simulink model "g1_G2_01"  (R2024a)
settings: Solver=ode1  StartTime=0.0  StopTime=0.3  FixedStep=Ts  RelTol=1e-3
PostLoadFcn:
  | GL_cbfcn('PostLoadFcn');
InitFcn:
  | GL_cbfcn('InitFcn');
StartFcn:
  | GL_cbfcn('StartFcn');
values from neighbouring files (symbols this model uses):
  Ts = 5e-4    (= 0.0005)    [g1_ini_01.m]    (also in g1_opam_ini_01.m; test.m = 0.001)
undefined symbols (not defined in the file or in its folder): burblks, DiscIntNeverNeededParam, GL_cbfcn
libraries: bur_blks x1
(part 1 of 2)
PreSaveFcn:
  | GL_cbfcn('PreSaveFcn');
PostSaveFcn:
  | GL_cbfcn('PostSaveFcn');
CloseFcn:
  | GL_cbfcn('CloseFcn');
settings Model: GhostLab=GhostLab  GhostLab_ModelName=Modular2  GhostLab_Version=2.0.4  CheckSum_Model=3251361011_3166437564_2525209146_3089150091  AS_Version=1.0.4  ExtModeTrigDuration=10000000  Creator=fldr  LastModifiedBy=rueegan5
settings DataIOCC: SaveFormat=Array  SaveOutput=off  SignalLogging=off  DSMLogging=off  SaveTime=off  ReturnWorkspaceOutputs=off
settings OptimizationCC: OptimizeBlockIOStorage=off  BufferReuse=off  GlobalBufferReuse=off  ExpressionFolding=off  EnableMemcpy=off  LocalBlockOutputs=off  InitFltsAndDblsToZero=on  LifeSpan=inf  OptimizeDataStoreBuffers=off  BusAssignmentInplaceUpdate=off
settings DebuggingCC: SaveWithDisabledLinksMsg=none  UnderspecifiedInitializationDetection=Classic  MergeDetectMultiDrivingBlocksExec=none  SolverPrmCheckMsg=warning  InheritedTsInSrcMsg=none  FcnCallInpInsideContextMsg=warning  FrameProcessingCompatibilityMsg=none  ModelReferenceSymbolNameMessage=none  StateNameClashWarn=warning  SFUnexpectedBacktrackingDiag=warning  SFNoUnconditionalDefaultTransitionDiag=warning
settings HardwareCC: ProdBitPerPointer=32  ProdBitPerSizeT=32  ProdBitPerPtrDiffT=32  ProdLargestAtomicFloat=None  ProdWordSize=32  ProdHWDeviceType=Intel->x86/Pentium
settings ModelReferenceCC: UpdateModelReferenceTargets=IfOutOfDate  ModelReferencePassRootInputsByReference=off  PropagateSignalLabelsOutOfModel=off
settings RTWCC: Description=B&R Automation Studio Target (GRT based)  SystemTargetFile=bur_grt.tlc  GenerateMakefile=off  TemplateMakefile=bur.tmf  RTWVerbose=off
settings RTWCC: CustomInitializer=|
  | udCheckSum0 = (0123456789U);
  | udCheckSum1 = (0123456789U);
  | udCheckSum2 = (0123456789U);
  | udCheckSum3 = (0123456789U);
  | udCurrentTime = &g1_G2_01_M->Timing.t[0];
  | udclockTick0 = &g1_G2_01_M->Timing.clockTick0;
  | udclockTickH0 = &g1_G2_01_M->Timing.clockTickH0;
  | udParam = &g1_G2_01_P;
  | udContinuousStates = &g1_G2_01_X;
  | udDiscreteStates = &g1_G2_01_DW;
settings CodeAppCC: MaxIdLength=255
settings STFCustomTargetCC: TargetLangStandard=C89/C90 (ANSI)  ParMdlRefBuildCompliant=on  UseToolchainInfoCompliant=off  SystemTargetFile=bur_grt.tlc
settings GRTTargetCC: TargetLangStandard=C89/C90 (ANSI)  CompOptLevelCompliant=off  ConcurrentExecutionCompliant=off  CombineOutputUpdateFcns=off  MatFileLogging=off  CPPClassGenCompliant=off  GRTInterface=on  UseToolchainInfoCompliant=off  ExtModeMexArgs='127.0.0.1'

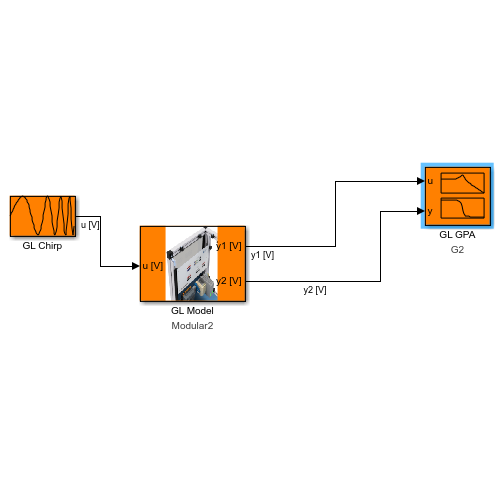
[thumbnail: Simulink's stored preview of the top-level diagram]
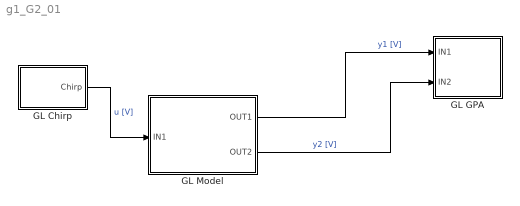
== system g1_G2_01 ==
  GL Chirp : Subsystem  LoadFcn=GL_cbfcn('loadChirp');  InitFcn=GL_cbfcn('initChirp');  mask(GhostLab Chirp){mode=logarithmic, f1=0.1, f2=1000, ampl=1, offs=0, T0=0, Tm=10, editSweepTime=off, Trig=1, mode_n=2, Dummy=0}
      mask prompts: mode "Sweep Sine Mode"; f1 "Start Frequency [Hz]"; f2 "End Frequency [Hz]"; ampl "Amplitude"; offs "Offset"; T0 "Settle Time [s]"; Tm "Sweep Time [s]"; editSweepTime "Edit"; Trig "Trigger"; mode_n "Chirp Mode"
      mask help: Creates a chirp (sweep sinus) signal used for gain phase analyzer.
      settings: CopyFcn=GL_cbfcn('copyChirp');  PreCopyFcn=GL_cbfcn('PreCopyChirp');
      mask Help: 1.0.2
      mask TypeOptions mode: linear | logarithmic | quadratic
      mask Callback mode:
      | try
      |     GL_cbfcn('ChirpMode');
      | end
      mask Callback f1:
      | try
      |     GL_cbfcn('fstart');
      | end
      | try
      |     GL_cbfcn('editSweepTime');
      | end
      mask Callback f2:
      | try
      |     GL_cbfcn('fend');
      | end
      mask Callback ampl:
      | try
      |     GL_cbfcn('ApplyChanges');
      | end
      mask Callback offs:
      | try
      |     GL_cbfcn('ApplyChanges');
      | end
      mask Callback T0:
      | try
      |     GL_cbfcn('ApplyChanges');
      | end
      mask Callback Tm:
      | try
      |     GL_cbfcn('ApplyChanges');
      | end
      mask Callback editSweepTime:
      | try
      |     GL_cbfcn('editSweepTime');
      | end
      mask DialogControl DescGroupVar Prompt: Chirp Signal Generator
      mask Display: plot(chirp(0:0.1:10,0.1,10,1,'logarithmic',-90));
  GL GPA : Subsystem  Tag=G2  Description=GL_cbfcn('openMask');  mask(GhostLab GPA){varname=G2}
      mask prompts: varname "Workspace Variable Name:"
      mask help:
      | Calculate and plot bode diagram using tfestimate.
      | An FRD-object and a structure with time data variable will be created in worspace.
      settings: AttributesFormatString=%<Tag>  CopyFcn=GL_cbfcn('copyGPA',gcb,'G');  DeleteFcn=GL_cbfcn('deleteScope');  UndoDeleteFcn=GL_cbfcn('updateScope');  PreCopyFcn=GL_cbfcn('PreCopyGPA');  OpenFcn=GL_cbfcn('openMask');
      mask Help: 1.0.2
      mask Callback varname: GL_cbfcn('set_var_name');
      mask DialogControl DescGroupVar Prompt: Gain Phase Analyzer
      mask DialogControl Control2 Prompt: help tfetimate
      mask DialogControl Control2 Callback: doc('tfestimate');
      mask DialogControl Container2 Prompt: Frequency Response Data (FRD) object:
      mask Display:
      | mat = [
      |    10.0000   78.3832   42.8007
      |    11.6327   78.3936   42.7806
      |    13.2653   78.4061   42.7584
      |    14.8980   78.4213   42.7338
      |    16.5306   78.4397   42.7064
      |    18.1633   78.4620   42.6761
      |    19.7959   78.4890   42.6423
      |    21.4286   78.5217   42.6044
      |    23.0612   78.5616   42.5620
      |    24.6939   78.6100   42.5142
      |    26.3265   78.6691   42.4600
      |    27.9592   78.7412   42.3982
      |    29.5918   78.8296   42.3272
      |    31.2245   78.9383   42.2447
      |    32.8571   79.0724   42.1478
      |    34.4898   79.2389   42.0322
      |    36.1224   79.4469   41.8917
      |    37.7551   79.7090   41.7169
      |    39.3878   80.0430   41.4928
      |    41.0204   80.4749   41.1939
      |    42.6531   81.0442   40.7735
      |    44.2857   81.8142   40.1368
      |    45.9184   82.8890   39.0620
      |    47.5510   84.4186   36.9274
      |    49.1837   86.2203   31.8362
      |    50.8163   85.7441   23.1638
      |    52.4490   82.9900   18.0726
      |    54.0816   80.5081   15.9380
      |    55.7143   78.4809   14.8632
      |    57.3469   76.7585   14.2265
      |    58.9796   75.2368   13.8061
      |    60.6122   73.8525   13.5072
      |    62.2449   72.5661   13.2831
      |    63.8776   71.3516   13.1083
      |    65.5102   70.1913   12.9678
      |    67.1429   69.0724   12.8522
      |    68.7755   67.9859   12.7553
      |    70.4082   66.9248   12.6728
      |    72.0408   65.8841   12.6018
      |    73.6735   64.8595   12.5400
      |    75.3061   63.8481   12.4858
      |    76.9388   62.8473   12.4380
      |    78.5714   61.8551   12.3956
      |    80.2041   60.8699   12.3577
      |    81.8367   59.8905   12.3239
      |    83.4694   58.9159   12.2936
      |    85.1020   57.9451   12.2662
      |    86.7347   56.9776   12.2416
      |    88.3673   56.0126   12.2194
      |    90.0000   55.0499   12.1993
      | ];
      | plot(-20,0,...
      |     100,100,...
      |     [10,90,90,10,10], [45,45,10,10,45],...
      |     [10,90,90,10,10], [90,90,55,55,90],...
      |     mat(:,1),mat(:,2),mat(:,1),mat(:,3));
      | port_label('input', 1, 'u');
      | port_label('input', 2, 'y');
  GL Model : Subsystem  Tag=Modular2  Description=GL_SetupModel;  mask(GhostLab Model){}
      settings: AttributesFormatString=%<Tag>  CopyFcn=GL_CopyFcn;  DeleteFcn=GL_cbfcn('Blk_DeleteFcn');  UndoDeleteFcn=GL_CopyFcn('BoW');  PreCopyFcn=GL_cbfcn('Blk_PreCopyFcn');  OpenFcn=GL_SetupModel;
      mask Display: image('Modular2.png',[0.25,0,0.5,1]);color('black');port_label('input', 1, 'u [V]');port_label('output', 1, 'y1 [V]');port_label('output', 2, 'y2 [V]');
  wires:
  GL Chirp/1(Chirp) -> GL Model/1(IN1)  "u [V]"
  GL Model/1(OUT1) -> GL GPA/1(IN1)  "y1 [V]"
  GL Model/2(OUT2) -> GL GPA/2(IN2)  "y2 [V]"

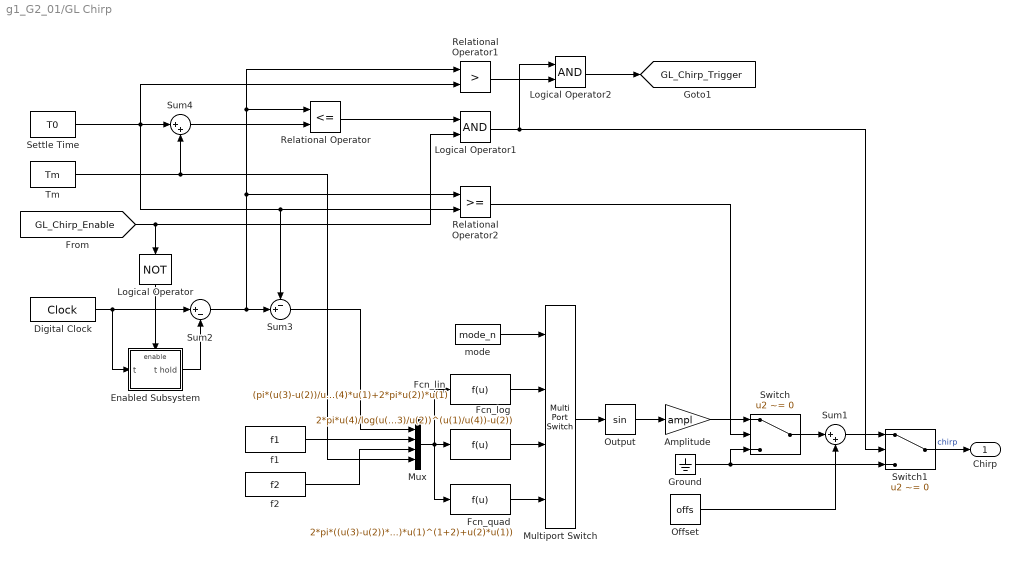
== system g1_G2_01/GL Chirp ==
  Amplitude : Gain  Gain=ampl
  Digital Clock : DigitalClock  SampleTime=Ts
  Enabled Subsystem : Subsystem  TreatAsAtomicUnit=on
  Fcn_lin : Fcn  Expr=(pi*(u(3)-u(2))/u(4)*u(1)+2*pi*u(2))*u(1)
  Fcn_log : Fcn  Expr=2*pi*u(4)/log(u(3)/u(2))*(u(2)*(u(3)/u(2))^(u(1)/u(4))-u(2))
  Fcn_quad : Fcn  Expr=2*pi*((u(3)-u(2))*u(4)^(-2)/(1+2)*u(1)^(1+2)+u(2)*u(1))
  Ground : Ground
  Logical Operator : Logic  Operator=NOT  AllPortsSameDT=off  OutDataTypeStr=boolean
  Logical Operator1 : Logic  AllPortsSameDT=off
  Logical Operator2 : Logic  AllPortsSameDT=off  OutDataTypeStr=boolean
  Multiport Switch : MultiPortSwitch  SaturateOnIntegerOverflow=off  InputSameDT=off
  Mux : Mux
  Offset : Constant  Value=offs
  Output : Trigonometry
  Relational Operator : RelationalOperator  Operator=<=  RndMeth=Simplest  InputSameDT=off
  Relational Operator1 : RelationalOperator  Operator=>  RndMeth=Simplest  InputSameDT=off
  Relational Operator2 : RelationalOperator  RndMeth=Simplest  InputSameDT=off
  Settle Time : Constant  Value=T0
  Sum1 : Sum  Inputs=|++
  Sum2 : Sum  Inputs=|+-
  Sum3 : Sum  Inputs=-+|
  Sum4 : Sum  Inputs=|++
  Switch : Switch  Criteria=u2 ~= 0  SaturateOnIntegerOverflow=off  InputSameDT=off
  Switch1 : Switch  Criteria=u2 ~= 0  SaturateOnIntegerOverflow=off  InputSameDT=off
  Tm : Constant  Value=Tm
  f1 : Constant  Value=f1
  f2 : Constant  Value=f2
  mode : Constant  Value=mode_n
  Chirp : Outport  VectorParamsAs1DForOutWhenUnconnected=off
  tag scope: GL_Chirp_Trigger=global
  wires:
  Relational Operator2/1 -> Switch/2
  Settle Time/1 -> Sum4/1, Relational Operator2/2, Sum3/1, Relational Operator1/2
  Sum4/1 -> Relational Operator/2
  Logical Operator/1 -> Enabled Subsystem/Enable
  Enabled Subsystem/1(t hold) -> Sum2/2
  [GL_Chirp_Enable] -> Logical Operator1/2, Logical Operator/1
  mode/1 -> Multiport Switch/1
  Fcn_lin/1 -> Multiport Switch/2
  Fcn_log/1 -> Multiport Switch/3
  Fcn_quad/1 -> Multiport Switch/4
  Multiport Switch/1 -> Output/1
  f2/1 -> Mux/3
  f1/1 -> Mux/2
  Mux/1 -> Fcn_log/1, Fcn_lin/1, Fcn_quad/1
  Output/1 -> Amplitude/1
  Offset/1 -> Sum1/2
  Sum3/1 -> Mux/1
  Tm/1 -> Sum4/2, Mux/4
  Switch/1 -> Sum1/1
  Amplitude/1 -> Switch/1
  Ground/1 -> Switch1/3, Switch/3
  Sum2/1 -> Relational Operator1/1, Relational Operator/1, Relational Operator2/1, Sum3/2
  Switch1/1 -> Chirp/1  "chirp"
  Sum1/1 -> Switch1/1
  Relational Operator/1 -> Logical Operator1/1
  Logical Operator1/1 -> Logical Operator2/1, Switch1/2
  Logical Operator2/1 -> [GL_Chirp_Trigger]
  Relational Operator1/1 -> Logical Operator2/2
  Digital Clock/1 -> Enabled Subsystem/1(t), Sum2/1

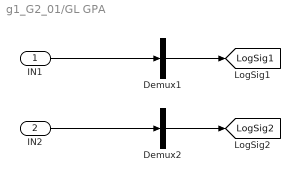
== system g1_G2_01/GL GPA ==
  IN1 : Inport
  IN2 : Inport  Port=2
  Demux1 : Demux  Outputs=1
  Demux2 : Demux  Outputs=1
  tag scope: LogSig1=global, LogSig2=global
  wires:
  IN2/1 -> Demux2/1
  IN1/1 -> Demux1/1
  Demux1/1 -> [LogSig1]
  Demux2/1 -> [LogSig2]

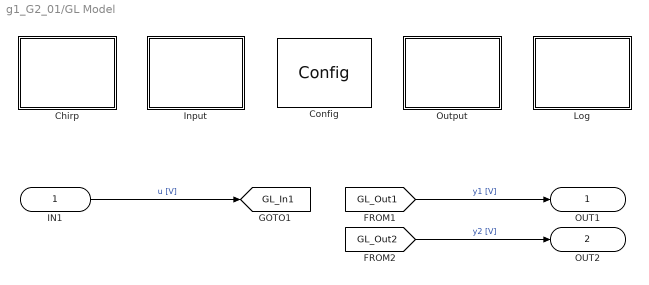
== system g1_G2_01/GL Model ==
  IN1 : Inport
  Chirp : Subsystem
  Config : bur_blks/Config  Tag=Coder: GRT C Target: Task  Description=burblks.classes.blks.BR_ConfigBlock.Do('open', gcb);  bur_configset_ert=C - Code Generation (Embedded Real Time Target based)  bur_configset_grt=C - Code Generation (Generic Real Time Target based)  bur_maskHandle=-1
      settings: AttributesFormatString=%<Tag>  SourceProductName=B&R Automation Studio Toolbox
  Input : Subsystem
  Log : Subsystem
  Output : Subsystem
  OUT1 : Outport
  OUT2 : Outport  Port=2
  tag scope: GL_In1=global
  wires:
  IN1/1 -> [GL_In1]  "u [V]"
  [GL_Out1] -> OUT1/1  "y1 [V]"
  [GL_Out2] -> OUT2/1  "y2 [V]"

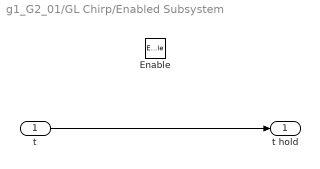
== system g1_G2_01/GL Chirp/Enabled Subsystem ==
  t : Inport
  Enable : EnablePort
  t hold : Outport  VectorParamsAs1DForOutWhenUnconnected=off
  wires:
  t/1 -> t hold/1

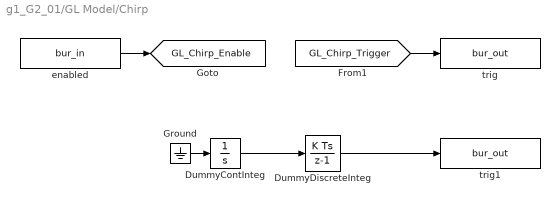
== system g1_G2_01/GL Model/Chirp ==
  DummyContInteg : Integrator
  DummyDiscreteInteg : DiscreteIntegrator  SampleTime=-1  OutDataTypeStr=single  ICPrevOutput=DiscIntNeverNeededParam  ICPrevScaledInput=DiscIntNeverNeededParam
  Ground : Ground
  enabled : S-Function  Tag=GLOBAL BOOL bConnectionEstablished  Description=burblks.classes.blks.BR_InputBlock.Do('open', gcb)  LoadFcn=burblks.classes.blks.BR_InputBlock.Do( 'load', gcb)  InitFcn=burblks.classes.blks.BR_InputBlock.Do('init', gcb)  FunctionName=bur_in  Parameters=bur_scope, bur_data_type, bur_init_value, bur_init_value_bool, bur_array_index, bur_var_name, bur_AS_string  SFunctionDeploymentMode=off  EnableBusSupport=off  mask(B&&R - Input Block){bur_var_name=bConnectionEstablished, bur_var_description=, bur_scope=GLOBAL, bur_data_type=BOOL, bur_init_value=0, bur_init_value_bool=FALSE, bur_array_index=0, bur_old_var_name=, bur_var_memory=standard, bur_in_parameter=off, bur_AS_string=bConnectionEstablished : BOOL := 0; (**), bur_array_index_string=0}
      mask prompts: bur_var_name "Variable Name"; bur_var_description "Variable Description"; bur_scope "Variable Scope"; bur_data_type "Variable Data Type"; bur_init_value "Initial Value"; bur_init_value_bool "Initial Value"; bur_array_index "Array Dimension (0...Scalar)"; bur_old_var_name "Old Variable Name"; bur_var_memory "Memory"; bur_in_parameter "Parameter"; bur_array_index_string "Array Dimension Variable (0..Scalar)"
      mask help: Input interface for B&R Automation Studio process variable.
      settings: AttributesFormatString=%<Tag>  CopyFcn=burblks.classes.blks.BR_InputBlock.Do('copy', gcb)  DeleteFcn=burblks.classes.blks.BR_InputBlock.Do( 'delete', gcb)  ModelCloseFcn=burblks.classes.blks.BR_InputBlock.Do('close', gcb)  PreSaveFcn=burblks.classes.blks.BR_InputBlock.Do('preSave', gcb)  PostSaveFcn=burblks.classes.blks.BR_InputBlock.Do('postSave', gcb)  OpenFcn=burblks.classes.blks.BR_InputBlock.Do('open', gcb)
      mask Help: eval('burblks.classes.blks.BR_BlockHelp.Help(''InputBlock'')')
      mask TypeOptions bur_scope: GLOBAL | LOCAL
      mask TypeOptions bur_data_type: LREAL | REAL | SINT | USINT | INT | UINT | DINT | UDINT | BOOL | STRING
      mask TypeOptions bur_init_value_bool: FALSE | TRUE
      mask TypeOptions bur_var_memory: standard | retain
      mask Display: color('orange'); disp('B&R IN');
  trig : S-Function  Tag=GLOBAL BOOL bGPAtrigger  Description=burblks.classes.blks.BR_OutputBlock.Do('open', gcb)  LoadFcn=burblks.classes.blks.BR_OutputBlock.Do( 'load', gcb)  InitFcn=burblks.classes.blks.BR_OutputBlock.Do('init', gcb)  FunctionName=bur_out  Parameters=bur_scope, bur_data_type, bur_init_value, bur_init_value_bool, bur_array_index, bur_var_name, bur_AS_string  SFunctionDeploymentMode=off  EnableBusSupport=off  mask(B&&R - Output Block){bur_var_name=bGPAtrigger, bur_var_description=, bur_scope=GLOBAL, bur_data_type=BOOL, bur_init_value=0, bur_init_value_bool=FALSE, bur_array_index=0, bur_old_var_name=, bur_var_memory=standard, bur_AS_string=bGPAtrigger : BOOL := 0; (**), bur_array_index_string=0}
      mask prompts: bur_var_name "Variable Name"; bur_var_description "Variable Description"; bur_scope "Variable Scope"; bur_data_type "Variable Data Type"; bur_init_value "Initial Value"; bur_init_value_bool "Initial Value"; bur_array_index "Array Dimension (0...Scalar)"; bur_old_var_name "Old Variable Name"; bur_var_memory "Memory"; bur_array_index_string "Array Dimension Variable (0..Scalar)"
      mask help: Output interface for B&R Automation Studio process variable.
      settings: AttributesFormatString=%<Tag>  CopyFcn=burblks.classes.blks.BR_OutputBlock.Do('copy', gcb)  DeleteFcn=burblks.classes.blks.BR_OutputBlock.Do( 'delete', gcb)  ModelCloseFcn=burblks.classes.blks.BR_OutputBlock.Do('close', gcb)  PreSaveFcn=burblks.classes.blks.BR_OutputBlock.Do('preSave', gcb)  PostSaveFcn=burblks.classes.blks.BR_OutputBlock.Do('postSave', gcb)  OpenFcn=burblks.classes.blks.BR_OutputBlock.Do('open', gcb)
      mask Help: eval('burblks.classes.blks.BR_BlockHelp.Help(''OutputBlock'')')
      mask TypeOptions bur_scope: GLOBAL | LOCAL
      mask TypeOptions bur_data_type: LREAL | REAL | SINT | USINT | INT | UINT | DINT | UDINT | BOOL | STRING
      mask TypeOptions bur_init_value_bool: FALSE | TRUE
      mask TypeOptions bur_var_memory: standard | retain
      mask Display: color('orange'); disp('B&R OUT');
  trig1 : S-Function  Tag=GLOBAL REAL rDummy  Description=burblks.classes.blks.BR_OutputBlock.Do('open', gcb)  LoadFcn=burblks.classes.blks.BR_OutputBlock.Do( 'load', gcb)  InitFcn=burblks.classes.blks.BR_OutputBlock.Do('init', gcb)  FunctionName=bur_out  Parameters=bur_scope, bur_data_type, bur_init_value, bur_init_value_bool, bur_array_index, bur_var_name, bur_AS_string  SFunctionDeploymentMode=off  EnableBusSupport=off  mask(B&&R - Output Block){bur_var_name=rDummy, bur_var_description=, bur_scope=GLOBAL, bur_data_type=REAL, bur_init_value=0, bur_init_value_bool=FALSE, bur_array_index=0, bur_old_var_name=, bur_var_memory=standard, bur_AS_string=rDummy : REAL := 0; (**), bur_array_index_string=0}
      mask prompts: bur_var_name "Variable Name"; bur_var_description "Variable Description"; bur_scope "Variable Scope"; bur_data_type "Variable Data Type"; bur_init_value "Initial Value"; bur_init_value_bool "Initial Value"; bur_array_index "Array Dimension (0...Scalar)"; bur_old_var_name "Old Variable Name"; bur_var_memory "Memory"; bur_array_index_string "Array Dimension Variable (0..Scalar)"
      mask help: Output interface for B&R Automation Studio process variable.
      settings: AttributesFormatString=%<Tag>  CopyFcn=burblks.classes.blks.BR_OutputBlock.Do('copy', gcb)  DeleteFcn=burblks.classes.blks.BR_OutputBlock.Do( 'delete', gcb)  ModelCloseFcn=burblks.classes.blks.BR_OutputBlock.Do('close', gcb)  PreSaveFcn=burblks.classes.blks.BR_OutputBlock.Do('preSave', gcb)  PostSaveFcn=burblks.classes.blks.BR_OutputBlock.Do('postSave', gcb)  OpenFcn=burblks.classes.blks.BR_OutputBlock.Do('open', gcb)
      mask Help: eval('burblks.classes.blks.BR_BlockHelp.Help(''OutputBlock'')')
      mask TypeOptions bur_scope: GLOBAL | LOCAL
      mask TypeOptions bur_data_type: LREAL | REAL | SINT | USINT | INT | UINT | DINT | UDINT | BOOL | STRING
      mask TypeOptions bur_init_value_bool: FALSE | TRUE
      mask TypeOptions bur_var_memory: standard | retain
      mask Display: color('orange'); disp('B&R OUT');
  tag scope: GL_Chirp_Enable=global
  wires:
  [GL_Chirp_Trigger] -> trig/1
  enabled/1 -> [GL_Chirp_Enable]
  DummyContInteg/1 -> DummyDiscreteInteg/1
  Ground/1 -> DummyContInteg/1
  DummyDiscreteInteg/1 -> trig1/1

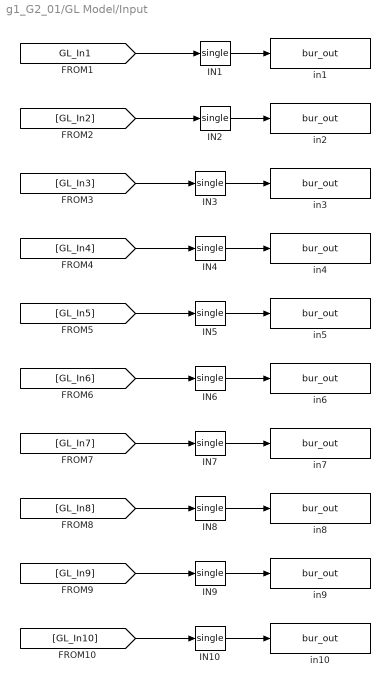
== system g1_G2_01/GL Model/Input ==
  IN{1..10} (10 alike) : DataTypeConversion  OutDataTypeStr=single  SaturateOnIntegerOverflow=off  RndMeth=Floor
  in1 : S-Function  Tag=GLOBAL REAL rSimInput1  Description=burblks.classes.blks.BR_OutputBlock.Do('open', gcb)  LoadFcn=burblks.classes.blks.BR_OutputBlock.Do( 'load', gcb)  InitFcn=burblks.classes.blks.BR_OutputBlock.Do('init', gcb)  FunctionName=bur_out  Parameters=bur_scope, bur_data_type, bur_init_value, bur_init_value_bool, bur_array_index, bur_var_name, bur_AS_string  SFunctionDeploymentMode=off  EnableBusSupport=off  mask(B&&R - Output Block){bur_var_name=rSimInput1, bur_var_description=, bur_scope=GLOBAL, bur_data_type=REAL, bur_init_value=0, bur_init_value_bool=FALSE, bur_array_index=0, bur_old_var_name=, bur_var_memory=standard, bur_AS_string=rSimInput1 : REAL := 0; (**), bur_array_index_string=0}
      mask prompts: bur_var_name "Variable Name"; bur_var_description "Variable Description"; bur_scope "Variable Scope"; bur_data_type "Variable Data Type"; bur_init_value "Initial Value"; bur_init_value_bool "Initial Value"; bur_array_index "Array Dimension (0...Scalar)"; bur_old_var_name "Old Variable Name"; bur_var_memory "Memory"; bur_array_index_string "Array Dimension Variable (0..Scalar)"
      mask help: Output interface for B&R Automation Studio process variable.
      settings: AttributesFormatString=%<Tag>  CopyFcn=burblks.classes.blks.BR_OutputBlock.Do('copy', gcb)  DeleteFcn=burblks.classes.blks.BR_OutputBlock.Do( 'delete', gcb)  ModelCloseFcn=burblks.classes.blks.BR_OutputBlock.Do('close', gcb)  PreSaveFcn=burblks.classes.blks.BR_OutputBlock.Do('preSave', gcb)  PostSaveFcn=burblks.classes.blks.BR_OutputBlock.Do('postSave', gcb)  OpenFcn=burblks.classes.blks.BR_OutputBlock.Do('open', gcb)
      mask Help: eval('burblks.classes.blks.BR_BlockHelp.Help(''OutputBlock'')')
      mask TypeOptions bur_scope: GLOBAL | LOCAL
      mask TypeOptions bur_data_type: LREAL | REAL | SINT | USINT | INT | UINT | DINT | UDINT | BOOL | STRING
      mask TypeOptions bur_init_value_bool: FALSE | TRUE
      mask TypeOptions bur_var_memory: standard | retain
      mask Display: color('orange'); disp('B&R OUT');
  in10 : S-Function  Tag=GLOBAL REAL rSimInput10  Description=burblks.classes.blks.BR_OutputBlock.Do('open', gcb)  LoadFcn=burblks.classes.blks.BR_OutputBlock.Do( 'load', gcb)  InitFcn=burblks.classes.blks.BR_OutputBlock.Do('init', gcb)  FunctionName=bur_out  Parameters=bur_scope, bur_data_type, bur_init_value, bur_init_value_bool, bur_array_index, bur_var_name, bur_AS_string  SFunctionDeploymentMode=off  EnableBusSupport=off  mask(B&&R - Output Block){bur_var_name=rSimInput10, bur_var_description=, bur_scope=GLOBAL, bur_data_type=REAL, bur_init_value=0, bur_init_value_bool=FALSE, bur_array_index=0, bur_old_var_name=, bur_var_memory=standard, bur_AS_string=rSimInput10 : REAL := 0; (**), bur_array_index_string=0}
      mask prompts: bur_var_name "Variable Name"; bur_var_description "Variable Description"; bur_scope "Variable Scope"; bur_data_type "Variable Data Type"; bur_init_value "Initial Value"; bur_init_value_bool "Initial Value"; bur_array_index "Array Dimension (0...Scalar)"; bur_old_var_name "Old Variable Name"; bur_var_memory "Memory"; bur_array_index_string "Array Dimension Variable (0..Scalar)"
      mask help: Output interface for B&R Automation Studio process variable.
      settings: AttributesFormatString=%<Tag>  CopyFcn=burblks.classes.blks.BR_OutputBlock.Do('copy', gcb)  DeleteFcn=burblks.classes.blks.BR_OutputBlock.Do( 'delete', gcb)  ModelCloseFcn=burblks.classes.blks.BR_OutputBlock.Do('close', gcb)  PreSaveFcn=burblks.classes.blks.BR_OutputBlock.Do('preSave', gcb)  PostSaveFcn=burblks.classes.blks.BR_OutputBlock.Do('postSave', gcb)  OpenFcn=burblks.classes.blks.BR_OutputBlock.Do('open', gcb)
      mask Help: eval('burblks.classes.blks.BR_BlockHelp.Help(''OutputBlock'')')
      mask TypeOptions bur_scope: GLOBAL | LOCAL
      mask TypeOptions bur_data_type: LREAL | REAL | SINT | USINT | INT | UINT | DINT | UDINT | BOOL | STRING
      mask TypeOptions bur_init_value_bool: FALSE | TRUE
      mask TypeOptions bur_var_memory: standard | retain
      mask Display: color('orange'); disp('B&R OUT');
  in2 : S-Function  Tag=GLOBAL REAL rSimInput2  Description=burblks.classes.blks.BR_OutputBlock.Do('open', gcb)  LoadFcn=burblks.classes.blks.BR_OutputBlock.Do( 'load', gcb)  InitFcn=burblks.classes.blks.BR_OutputBlock.Do('init', gcb)  FunctionName=bur_out  Parameters=bur_scope, bur_data_type, bur_init_value, bur_init_value_bool, bur_array_index, bur_var_name, bur_AS_string  SFunctionDeploymentMode=off  EnableBusSupport=off  mask(B&&R - Output Block){bur_var_name=rSimInput2, bur_var_description=, bur_scope=GLOBAL, bur_data_type=REAL, bur_init_value=0, bur_init_value_bool=FALSE, bur_array_index=0, bur_old_var_name=, bur_var_memory=standard, bur_AS_string=rSimInput2 : REAL := 0; (**), bur_array_index_string=0}
      mask prompts: bur_var_name "Variable Name"; bur_var_description "Variable Description"; bur_scope "Variable Scope"; bur_data_type "Variable Data Type"; bur_init_value "Initial Value"; bur_init_value_bool "Initial Value"; bur_array_index "Array Dimension (0...Scalar)"; bur_old_var_name "Old Variable Name"; bur_var_memory "Memory"; bur_array_index_string "Array Dimension Variable (0..Scalar)"
      mask help: Output interface for B&R Automation Studio process variable.
      settings: AttributesFormatString=%<Tag>  CopyFcn=burblks.classes.blks.BR_OutputBlock.Do('copy', gcb)  DeleteFcn=burblks.classes.blks.BR_OutputBlock.Do( 'delete', gcb)  ModelCloseFcn=burblks.classes.blks.BR_OutputBlock.Do('close', gcb)  PreSaveFcn=burblks.classes.blks.BR_OutputBlock.Do('preSave', gcb)  PostSaveFcn=burblks.classes.blks.BR_OutputBlock.Do('postSave', gcb)  OpenFcn=burblks.classes.blks.BR_OutputBlock.Do('open', gcb)
      mask Help: eval('burblks.classes.blks.BR_BlockHelp.Help(''OutputBlock'')')
      mask TypeOptions bur_scope: GLOBAL | LOCAL
      mask TypeOptions bur_data_type: LREAL | REAL | SINT | USINT | INT | UINT | DINT | UDINT | BOOL | STRING
      mask TypeOptions bur_init_value_bool: FALSE | TRUE
      mask TypeOptions bur_var_memory: standard | retain
      mask Display: color('orange'); disp('B&R OUT');
  in3 : S-Function  Tag=GLOBAL REAL rSimInput3  Description=burblks.classes.blks.BR_OutputBlock.Do('open', gcb)  LoadFcn=burblks.classes.blks.BR_OutputBlock.Do( 'load', gcb)  InitFcn=burblks.classes.blks.BR_OutputBlock.Do('init', gcb)  FunctionName=bur_out  Parameters=bur_scope, bur_data_type, bur_init_value, bur_init_value_bool, bur_array_index, bur_var_name, bur_AS_string  SFunctionDeploymentMode=off  EnableBusSupport=off  mask(B&&R - Output Block){bur_var_name=rSimInput3, bur_var_description=, bur_scope=GLOBAL, bur_data_type=REAL, bur_init_value=0, bur_init_value_bool=FALSE, bur_array_index=0, bur_old_var_name=, bur_var_memory=standard, bur_AS_string=rSimInput3 : REAL := 0; (**), bur_array_index_string=0}
      mask prompts: bur_var_name "Variable Name"; bur_var_description "Variable Description"; bur_scope "Variable Scope"; bur_data_type "Variable Data Type"; bur_init_value "Initial Value"; bur_init_value_bool "Initial Value"; bur_array_index "Array Dimension (0...Scalar)"; bur_old_var_name "Old Variable Name"; bur_var_memory "Memory"; bur_array_index_string "Array Dimension Variable (0..Scalar)"
      mask help: Output interface for B&R Automation Studio process variable.
      settings: AttributesFormatString=%<Tag>  CopyFcn=burblks.classes.blks.BR_OutputBlock.Do('copy', gcb)  DeleteFcn=burblks.classes.blks.BR_OutputBlock.Do( 'delete', gcb)  ModelCloseFcn=burblks.classes.blks.BR_OutputBlock.Do('close', gcb)  PreSaveFcn=burblks.classes.blks.BR_OutputBlock.Do('preSave', gcb)  PostSaveFcn=burblks.classes.blks.BR_OutputBlock.Do('postSave', gcb)  OpenFcn=burblks.classes.blks.BR_OutputBlock.Do('open', gcb)
      mask Help: eval('burblks.classes.blks.BR_BlockHelp.Help(''OutputBlock'')')
      mask TypeOptions bur_scope: GLOBAL | LOCAL
      mask TypeOptions bur_data_type: LREAL | REAL | SINT | USINT | INT | UINT | DINT | UDINT | BOOL | STRING
      mask TypeOptions bur_init_value_bool: FALSE | TRUE
      mask TypeOptions bur_var_memory: standard | retain
      mask Display: color('orange'); disp('B&R OUT');
  in4 : S-Function  Tag=GLOBAL REAL rSimInput4  Description=burblks.classes.blks.BR_OutputBlock.Do('open', gcb)  LoadFcn=burblks.classes.blks.BR_OutputBlock.Do( 'load', gcb)  InitFcn=burblks.classes.blks.BR_OutputBlock.Do('init', gcb)  FunctionName=bur_out  Parameters=bur_scope, bur_data_type, bur_init_value, bur_init_value_bool, bur_array_index, bur_var_name, bur_AS_string  SFunctionDeploymentMode=off  EnableBusSupport=off  mask(B&&R - Output Block){bur_var_name=rSimInput4, bur_var_description=, bur_scope=GLOBAL, bur_data_type=REAL, bur_init_value=0, bur_init_value_bool=FALSE, bur_array_index=0, bur_old_var_name=, bur_var_memory=standard, bur_AS_string=rSimInput4 : REAL := 0; (**), bur_array_index_string=0}
      mask prompts: bur_var_name "Variable Name"; bur_var_description "Variable Description"; bur_scope "Variable Scope"; bur_data_type "Variable Data Type"; bur_init_value "Initial Value"; bur_init_value_bool "Initial Value"; bur_array_index "Array Dimension (0...Scalar)"; bur_old_var_name "Old Variable Name"; bur_var_memory "Memory"; bur_array_index_string "Array Dimension Variable (0..Scalar)"
      mask help: Output interface for B&R Automation Studio process variable.
      settings: AttributesFormatString=%<Tag>  CopyFcn=burblks.classes.blks.BR_OutputBlock.Do('copy', gcb)  DeleteFcn=burblks.classes.blks.BR_OutputBlock.Do( 'delete', gcb)  ModelCloseFcn=burblks.classes.blks.BR_OutputBlock.Do('close', gcb)  PreSaveFcn=burblks.classes.blks.BR_OutputBlock.Do('preSave', gcb)  PostSaveFcn=burblks.classes.blks.BR_OutputBlock.Do('postSave', gcb)  OpenFcn=burblks.classes.blks.BR_OutputBlock.Do('open', gcb)
      mask Help: eval('burblks.classes.blks.BR_BlockHelp.Help(''OutputBlock'')')
      mask TypeOptions bur_scope: GLOBAL | LOCAL
      mask TypeOptions bur_data_type: LREAL | REAL | SINT | USINT | INT | UINT | DINT | UDINT | BOOL | STRING
      mask TypeOptions bur_init_value_bool: FALSE | TRUE
      mask TypeOptions bur_var_memory: standard | retain
      mask Display: color('orange'); disp('B&R OUT');
  in5 : S-Function  Tag=GLOBAL REAL rSimInput5  Description=burblks.classes.blks.BR_OutputBlock.Do('open', gcb)  LoadFcn=burblks.classes.blks.BR_OutputBlock.Do( 'load', gcb)  InitFcn=burblks.classes.blks.BR_OutputBlock.Do('init', gcb)  FunctionName=bur_out  Parameters=bur_scope, bur_data_type, bur_init_value, bur_init_value_bool, bur_array_index, bur_var_name, bur_AS_string  SFunctionDeploymentMode=off  EnableBusSupport=off  mask(B&&R - Output Block){bur_var_name=rSimInput5, bur_var_description=, bur_scope=GLOBAL, bur_data_type=REAL, bur_init_value=0, bur_init_value_bool=FALSE, bur_array_index=0, bur_old_var_name=, bur_var_memory=standard, bur_AS_string=rSimInput5 : REAL := 0; (**), bur_array_index_string=0}
      mask prompts: bur_var_name "Variable Name"; bur_var_description "Variable Description"; bur_scope "Variable Scope"; bur_data_type "Variable Data Type"; bur_init_value "Initial Value"; bur_init_value_bool "Initial Value"; bur_array_index "Array Dimension (0...Scalar)"; bur_old_var_name "Old Variable Name"; bur_var_memory "Memory"; bur_array_index_string "Array Dimension Variable (0..Scalar)"
      mask help: Output interface for B&R Automation Studio process variable.
      settings: AttributesFormatString=%<Tag>  CopyFcn=burblks.classes.blks.BR_OutputBlock.Do('copy', gcb)  DeleteFcn=burblks.classes.blks.BR_OutputBlock.Do( 'delete', gcb)  ModelCloseFcn=burblks.classes.blks.BR_OutputBlock.Do('close', gcb)  PreSaveFcn=burblks.classes.blks.BR_OutputBlock.Do('preSave', gcb)  PostSaveFcn=burblks.classes.blks.BR_OutputBlock.Do('postSave', gcb)  OpenFcn=burblks.classes.blks.BR_OutputBlock.Do('open', gcb)
      mask Help: eval('burblks.classes.blks.BR_BlockHelp.Help(''OutputBlock'')')
      mask TypeOptions bur_scope: GLOBAL | LOCAL
      mask TypeOptions bur_data_type: LREAL | REAL | SINT | USINT | INT | UINT | DINT | UDINT | BOOL | STRING
      mask TypeOptions bur_init_value_bool: FALSE | TRUE
      mask TypeOptions bur_var_memory: standard | retain
      mask Display: color('orange'); disp('B&R OUT');
  in6 : S-Function  Tag=GLOBAL REAL rSimInput6  Description=burblks.classes.blks.BR_OutputBlock.Do('open', gcb)  LoadFcn=burblks.classes.blks.BR_OutputBlock.Do( 'load', gcb)  InitFcn=burblks.classes.blks.BR_OutputBlock.Do('init', gcb)  FunctionName=bur_out  Parameters=bur_scope, bur_data_type, bur_init_value, bur_init_value_bool, bur_array_index, bur_var_name, bur_AS_string  SFunctionDeploymentMode=off  EnableBusSupport=off  mask(B&&R - Output Block){bur_var_name=rSimInput6, bur_var_description=, bur_scope=GLOBAL, bur_data_type=REAL, bur_init_value=0, bur_init_value_bool=FALSE, bur_array_index=0, bur_old_var_name=, bur_var_memory=standard, bur_AS_string=rSimInput6 : REAL := 0; (**), bur_array_index_string=0}
      mask prompts: bur_var_name "Variable Name"; bur_var_description "Variable Description"; bur_scope "Variable Scope"; bur_data_type "Variable Data Type"; bur_init_value "Initial Value"; bur_init_value_bool "Initial Value"; bur_array_index "Array Dimension (0...Scalar)"; bur_old_var_name "Old Variable Name"; bur_var_memory "Memory"; bur_array_index_string "Array Dimension Variable (0..Scalar)"
      mask help: Output interface for B&R Automation Studio process variable.
      settings: AttributesFormatString=%<Tag>  CopyFcn=burblks.classes.blks.BR_OutputBlock.Do('copy', gcb)  DeleteFcn=burblks.classes.blks.BR_OutputBlock.Do( 'delete', gcb)  ModelCloseFcn=burblks.classes.blks.BR_OutputBlock.Do('close', gcb)  PreSaveFcn=burblks.classes.blks.BR_OutputBlock.Do('preSave', gcb)  PostSaveFcn=burblks.classes.blks.BR_OutputBlock.Do('postSave', gcb)  OpenFcn=burblks.classes.blks.BR_OutputBlock.Do('open', gcb)
      mask Help: eval('burblks.classes.blks.BR_BlockHelp.Help(''OutputBlock'')')
      mask TypeOptions bur_scope: GLOBAL | LOCAL
      mask TypeOptions bur_data_type: LREAL | REAL | SINT | USINT | INT | UINT | DINT | UDINT | BOOL | STRING
      mask TypeOptions bur_init_value_bool: FALSE | TRUE
      mask TypeOptions bur_var_memory: standard | retain
      mask Display: color('orange'); disp('B&R OUT');
  in7 : S-Function  Tag=GLOBAL REAL rSimInput7  Description=burblks.classes.blks.BR_OutputBlock.Do('open', gcb)  LoadFcn=burblks.classes.blks.BR_OutputBlock.Do( 'load', gcb)  InitFcn=burblks.classes.blks.BR_OutputBlock.Do('init', gcb)  FunctionName=bur_out  Parameters=bur_scope, bur_data_type, bur_init_value, bur_init_value_bool, bur_array_index, bur_var_name, bur_AS_string  SFunctionDeploymentMode=off  EnableBusSupport=off  mask(B&&R - Output Block){bur_var_name=rSimInput7, bur_var_description=, bur_scope=GLOBAL, bur_data_type=REAL, bur_init_value=0, bur_init_value_bool=FALSE, bur_array_index=0, bur_old_var_name=, bur_var_memory=standard, bur_AS_string=rSimInput7 : REAL := 0; (**), bur_array_index_string=0}
      mask prompts: bur_var_name "Variable Name"; bur_var_description "Variable Description"; bur_scope "Variable Scope"; bur_data_type "Variable Data Type"; bur_init_value "Initial Value"; bur_init_value_bool "Initial Value"; bur_array_index "Array Dimension (0...Scalar)"; bur_old_var_name "Old Variable Name"; bur_var_memory "Memory"; bur_array_index_string "Array Dimension Variable (0..Scalar)"
      mask help: Output interface for B&R Automation Studio process variable.
      settings: AttributesFormatString=%<Tag>  CopyFcn=burblks.classes.blks.BR_OutputBlock.Do('copy', gcb)  DeleteFcn=burblks.classes.blks.BR_OutputBlock.Do( 'delete', gcb)  ModelCloseFcn=burblks.classes.blks.BR_OutputBlock.Do('close', gcb)  PreSaveFcn=burblks.classes.blks.BR_OutputBlock.Do('preSave', gcb)  PostSaveFcn=burblks.classes.blks.BR_OutputBlock.Do('postSave', gcb)  OpenFcn=burblks.classes.blks.BR_OutputBlock.Do('open', gcb)
      mask Help: eval('burblks.classes.blks.BR_BlockHelp.Help(''OutputBlock'')')
      mask TypeOptions bur_scope: GLOBAL | LOCAL
      mask TypeOptions bur_data_type: LREAL | REAL | SINT | USINT | INT | UINT | DINT | UDINT | BOOL | STRING
      mask TypeOptions bur_init_value_bool: FALSE | TRUE
      mask TypeOptions bur_var_memory: standard | retain
      mask Display: color('orange'); disp('B&R OUT');
  in8 : S-Function  Tag=GLOBAL REAL rSimInput8  Description=burblks.classes.blks.BR_OutputBlock.Do('open', gcb)  LoadFcn=burblks.classes.blks.BR_OutputBlock.Do( 'load', gcb)  InitFcn=burblks.classes.blks.BR_OutputBlock.Do('init', gcb)  FunctionName=bur_out  Parameters=bur_scope, bur_data_type, bur_init_value, bur_init_value_bool, bur_array_index, bur_var_name, bur_AS_string  SFunctionDeploymentMode=off  EnableBusSupport=off  mask(B&&R - Output Block){bur_var_name=rSimInput8, bur_var_description=, bur_scope=GLOBAL, bur_data_type=REAL, bur_init_value=0, bur_init_value_bool=FALSE, bur_array_index=0, bur_old_var_name=, bur_var_memory=standard, bur_AS_string=rSimInput8 : REAL := 0; (**), bur_array_index_string=0}
      mask prompts: bur_var_name "Variable Name"; bur_var_description "Variable Description"; bur_scope "Variable Scope"; bur_data_type "Variable Data Type"; bur_init_value "Initial Value"; bur_init_value_bool "Initial Value"; bur_array_index "Array Dimension (0...Scalar)"; bur_old_var_name "Old Variable Name"; bur_var_memory "Memory"; bur_array_index_string "Array Dimension Variable (0..Scalar)"
      mask help: Output interface for B&R Automation Studio process variable.
      settings: AttributesFormatString=%<Tag>  CopyFcn=burblks.classes.blks.BR_OutputBlock.Do('copy', gcb)  DeleteFcn=burblks.classes.blks.BR_OutputBlock.Do( 'delete', gcb)  ModelCloseFcn=burblks.classes.blks.BR_OutputBlock.Do('close', gcb)  PreSaveFcn=burblks.classes.blks.BR_OutputBlock.Do('preSave', gcb)  PostSaveFcn=burblks.classes.blks.BR_OutputBlock.Do('postSave', gcb)  OpenFcn=burblks.classes.blks.BR_OutputBlock.Do('open', gcb)
      mask Help: eval('burblks.classes.blks.BR_BlockHelp.Help(''OutputBlock'')')
      mask TypeOptions bur_scope: GLOBAL | LOCAL
      mask TypeOptions bur_data_type: LREAL | REAL | SINT | USINT | INT | UINT | DINT | UDINT | BOOL | STRING
      mask TypeOptions bur_init_value_bool: FALSE | TRUE
      mask TypeOptions bur_var_memory: standard | retain
      mask Display: color('orange'); disp('B&R OUT');
  in9 : S-Function  Tag=GLOBAL REAL rSimInput9  Description=burblks.classes.blks.BR_OutputBlock.Do('open', gcb)  LoadFcn=burblks.classes.blks.BR_OutputBlock.Do( 'load', gcb)  InitFcn=burblks.classes.blks.BR_OutputBlock.Do('init', gcb)  FunctionName=bur_out  Parameters=bur_scope, bur_data_type, bur_init_value, bur_init_value_bool, bur_array_index, bur_var_name, bur_AS_string  SFunctionDeploymentMode=off  EnableBusSupport=off  mask(B&&R - Output Block){bur_var_name=rSimInput9, bur_var_description=, bur_scope=GLOBAL, bur_data_type=REAL, bur_init_value=0, bur_init_value_bool=FALSE, bur_array_index=0, bur_old_var_name=, bur_var_memory=standard, bur_AS_string=rSimInput9 : REAL := 0; (**), bur_array_index_string=0}
      mask prompts: bur_var_name "Variable Name"; bur_var_description "Variable Description"; bur_scope "Variable Scope"; bur_data_type "Variable Data Type"; bur_init_value "Initial Value"; bur_init_value_bool "Initial Value"; bur_array_index "Array Dimension (0...Scalar)"; bur_old_var_name "Old Variable Name"; bur_var_memory "Memory"; bur_array_index_string "Array Dimension Variable (0..Scalar)"
      mask help: Output interface for B&R Automation Studio process variable.
      settings: AttributesFormatString=%<Tag>  CopyFcn=burblks.classes.blks.BR_OutputBlock.Do('copy', gcb)  DeleteFcn=burblks.classes.blks.BR_OutputBlock.Do( 'delete', gcb)  ModelCloseFcn=burblks.classes.blks.BR_OutputBlock.Do('close', gcb)  PreSaveFcn=burblks.classes.blks.BR_OutputBlock.Do('preSave', gcb)  PostSaveFcn=burblks.classes.blks.BR_OutputBlock.Do('postSave', gcb)  OpenFcn=burblks.classes.blks.BR_OutputBlock.Do('open', gcb)
      mask Help: eval('burblks.classes.blks.BR_BlockHelp.Help(''OutputBlock'')')
      mask TypeOptions bur_scope: GLOBAL | LOCAL
      mask TypeOptions bur_data_type: LREAL | REAL | SINT | USINT | INT | UINT | DINT | UDINT | BOOL | STRING
      mask TypeOptions bur_init_value_bool: FALSE | TRUE
      mask TypeOptions bur_var_memory: standard | retain
      mask Display: color('orange'); disp('B&R OUT');
  wires:
  IN5/1 -> in5/1
  IN8/1 -> in8/1
  [GL_In8] -> IN8/1
  IN9/1 -> in9/1
  [GL_In9] -> IN9/1
  IN6/1 -> in6/1
  IN3/1 -> in3/1
  [GL_In5] -> IN5/1
  [GL_In3] -> IN3/1
  [GL_In1] -> IN1/1
  [GL_In6] -> IN6/1
  IN2/1 -> in2/1
  [GL_In4] -> IN4/1
  IN10/1 -> in10/1
  [GL_In7] -> IN7/1
  [GL_In10] -> IN10/1
  IN1/1 -> in1/1
  IN4/1 -> in4/1
  IN7/1 -> in7/1
  [GL_In2] -> IN2/1
